simulink model "netraScreeningThroughput"  (R2026a)
settings: Solver=VariableStepAuto
InitFcn:
  | addpath(fileparts(get_param(bdroot,'FileName'))); d = computeDerivedVariables(throughputParams()); ArrivalRateDuringHours = d.ArrivalRateDuringHours; ArrivalDutyCyclePercent = d.ArrivalDutyCyclePercent; TransmissionCapacity = d.TransmissionCapacity; ProcessingCapacity = d.ProcessingCapacity; ReferralRate = d.ReferralRate; ReviewCapacity = d.ReviewCapacity; clear d;
settings Model: Creator=aarav  LastModifiedBy=aarav

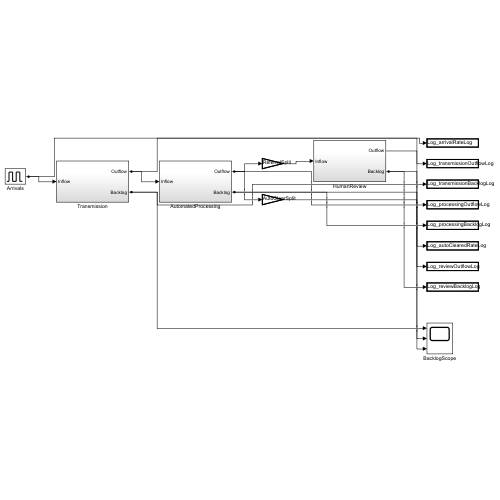
[thumbnail: Simulink's stored preview of the top-level diagram]
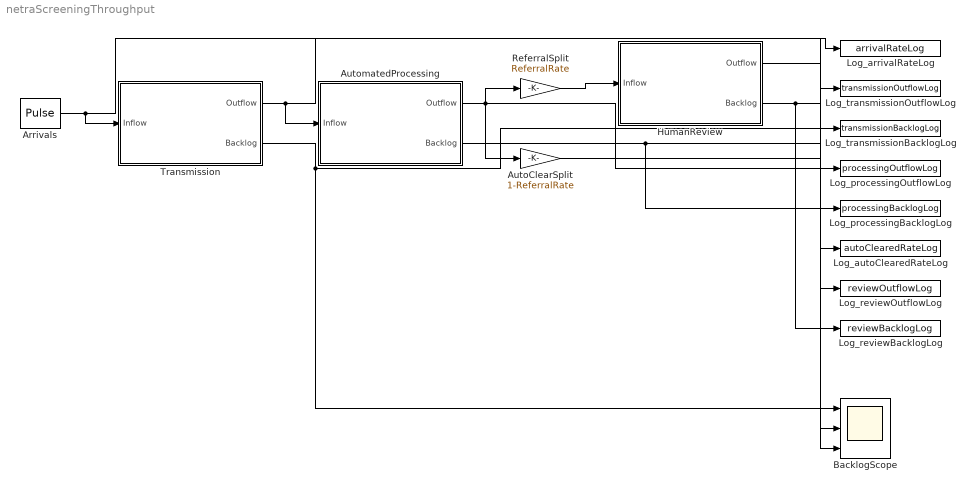
== system netraScreeningThroughput ==
  Arrivals : DiscretePulseGenerator  PulseType=Time based  Amplitude=ArrivalRateDuringHours  Period=24  PulseWidth=ArrivalDutyCyclePercent
  AutoClearSplit : Gain  Gain=1-ReferralRate
  AutomatedProcessing : Subsystem
  BacklogScope : Scope  NumInputPorts=3
  HumanReview : Subsystem
  Log_arrivalRateLog : ToWorkspace  VariableName=arrivalRateLog  SaveFormat=Structure With Time  SampleTime=-1
  Log_autoClearedRateLog : ToWorkspace  VariableName=autoClearedRateLog  SaveFormat=Structure With Time  SampleTime=-1
  Log_processingBacklogLog : ToWorkspace  VariableName=processingBacklogLog  SaveFormat=Structure With Time  SampleTime=-1
  Log_processingOutflowLog : ToWorkspace  VariableName=processingOutflowLog  SaveFormat=Structure With Time  SampleTime=-1
  Log_reviewBacklogLog : ToWorkspace  VariableName=reviewBacklogLog  SaveFormat=Structure With Time  SampleTime=-1
  Log_reviewOutflowLog : ToWorkspace  VariableName=reviewOutflowLog  SaveFormat=Structure With Time  SampleTime=-1
  Log_transmissionBacklogLog : ToWorkspace  VariableName=transmissionBacklogLog  SaveFormat=Structure With Time  SampleTime=-1
  Log_transmissionOutflowLog : ToWorkspace  VariableName=transmissionOutflowLog  SaveFormat=Structure With Time  SampleTime=-1
  ReferralSplit : Gain  Gain=ReferralRate
  Transmission : Subsystem
  wires:
  Transmission/2(Backlog) -> BacklogScope/1, Log_transmissionBacklogLog/1
  AutomatedProcessing/2(Backlog) -> BacklogScope/2, Log_processingBacklogLog/1
  HumanReview/2(Backlog) -> BacklogScope/3, Log_reviewBacklogLog/1
  Arrivals/1 -> Transmission/1(Inflow), Log_arrivalRateLog/1
  Transmission/1(Outflow) -> AutomatedProcessing/1(Inflow), Log_transmissionOutflowLog/1
  AutomatedProcessing/1(Outflow) -> ReferralSplit/1, AutoClearSplit/1, Log_processingOutflowLog/1
  ReferralSplit/1 -> HumanReview/1(Inflow)
  AutoClearSplit/1 -> Log_autoClearedRateLog/1
  HumanReview/1(Outflow) -> Log_reviewOutflowLog/1

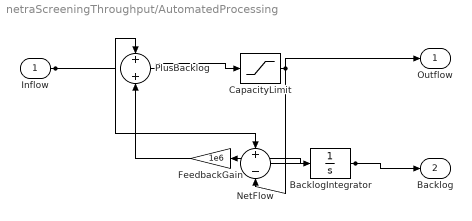
== system netraScreeningThroughput/AutomatedProcessing ==
  Inflow : Inport
  BacklogIntegrator : Integrator  LimitOutput=on  LowerSaturationLimit=0
  CapacityLimit : Saturate  UpperLimit=ProcessingCapacity  LowerLimit=0
  FeedbackGain : Gain  Gain=1e6
  NetFlow : Sum  Inputs=+-
  PlusBacklog : Sum
  Outflow : Outport
  Backlog : Outport  Port=2
  wires:
  ? -> ?
  Inflow/1 -> PlusBacklog/1, NetFlow/1
  PlusBacklog/1 -> CapacityLimit/1
  CapacityLimit/1 -> Outflow/1, NetFlow/2
  NetFlow/1 -> BacklogIntegrator/1
  BacklogIntegrator/1 -> Backlog/1, FeedbackGain/1
  FeedbackGain/1 -> PlusBacklog/2

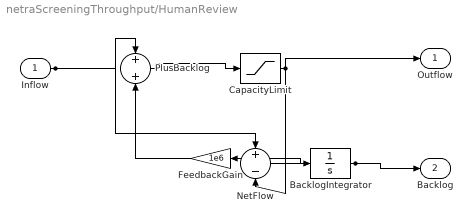
== system netraScreeningThroughput/HumanReview ==
  Inflow : Inport
  BacklogIntegrator : Integrator  LimitOutput=on  LowerSaturationLimit=0
  CapacityLimit : Saturate  UpperLimit=ReviewCapacity  LowerLimit=0
  FeedbackGain : Gain  Gain=1e6
  NetFlow : Sum  Inputs=+-
  PlusBacklog : Sum
  Outflow : Outport
  Backlog : Outport  Port=2
  wires:
  ? -> ?
  Inflow/1 -> PlusBacklog/1, NetFlow/1
  PlusBacklog/1 -> CapacityLimit/1
  CapacityLimit/1 -> Outflow/1, NetFlow/2
  NetFlow/1 -> BacklogIntegrator/1
  BacklogIntegrator/1 -> Backlog/1, FeedbackGain/1
  FeedbackGain/1 -> PlusBacklog/2

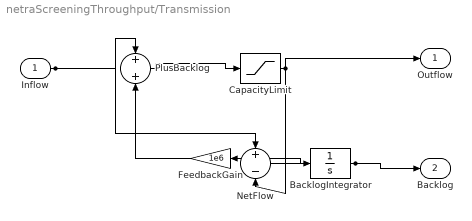
== system netraScreeningThroughput/Transmission ==
  Inflow : Inport
  BacklogIntegrator : Integrator  LimitOutput=on  LowerSaturationLimit=0
  CapacityLimit : Saturate  UpperLimit=TransmissionCapacity  LowerLimit=0
  FeedbackGain : Gain  Gain=1e6
  NetFlow : Sum  Inputs=+-
  PlusBacklog : Sum
  Outflow : Outport
  Backlog : Outport  Port=2
  wires:
  ? -> ?
  Inflow/1 -> PlusBacklog/1, NetFlow/1
  PlusBacklog/1 -> CapacityLimit/1
  CapacityLimit/1 -> Outflow/1, NetFlow/2
  NetFlow/1 -> BacklogIntegrator/1
  BacklogIntegrator/1 -> Backlog/1, FeedbackGain/1
  FeedbackGain/1 -> PlusBacklog/2
